simulink library "carnot"  (R2018b)
settings: Solver=VariableStepAuto  StartTime=0.0  StopTime=10.0  RelTol=1e-3
undefined symbols (not defined in the file or in its folder): A, A_earth, acol, Acol, ActPower1, ActPower2, ActPower3, Ad, Ad0, Ar, Au, Au0, Azimuth_Angle, B, Bd, Bd0, Br, Bu, Bu0, C, c1, c2, c3, c33, c4, c5, c6, CarnotCallbacks_Density, CarnotCallbacks_Enthalpy, CarnotCallbacks_Enthalpy2Temperature, CarnotCallbacks_Entropy, CarnotCallbacks_Evaporation_Enthalpy, CarnotCallbacks_GlobalMessageLevel, CarnotCallbacks_Grashof, CarnotCallbacks_Heat_Capacity, CarnotCallbacks_Kinematic_Viscosity, CarnotCallbacks_PMV_PPD, CarnotCallbacks_Prandtl, CarnotCallbacks_Saturation_Property, CarnotCallbacks_Saturation_Temperature, CarnotCallbacks_Saturation_Value_Water, CarnotCallbacks_Specific_Volume, CarnotCallbacks_Thermal_Conductivity, CarnotCallbacks_Vapour_Content, CarnotCallbacks_Vapour_Pressure, Cd, Cdl, Cr, Cu, Davies, Dd, DE_TRY2010_04_averageYear, delta_grd, density, DiameterLastPiece, dl, DPConstant, DPLinear, DPQuadratic, Dr ... (+59)
libraries: $bdroot x429, simulink x36, simulink_extras x12
(part 17 of 22)

== system carnot/Source/Solar_Thermal/IncidenceAngleModifier ==
  IAM_Table : Subsystem  mask(IAM Table for Solar Thermal Collectors){fta=0.8, angle=[0:5:90], Kb=[1.0000    1.0000    0.9999    0.9996    0.9991    0.9982    0.9965  0.9935    0.9886    0.9807    0.9678    0.9473    0.9148    0.8638   0.7846    0.6644    0.4907    0.2599    0.0000], Kd=0.92}
      mask prompts: fta "Fin Efficiency * Transmission * Absorption (FTA) [-]"; angle "Direct incidence angles for IAM [degree]"; Kb "Kdir: Incidence angle modifier direct radiation (0..1)"; Kd "Kdfu : Incidence angle modifier diffuse radiation"
      mask help:
      | Transforms direct and diffuse radiation to an absorbed solar power per unit area. The direct radiation incidence angle modifier (Kdir) uses the table-model for collectors (EN 12975).
      | FTA or F'(TauAlfa) is defined from the incidence angle modifiers Kdir and Kdfu:
      | FTA = eta0 / (Kdir(15°)*0.85 + Kdfu*0.15)
      | Direct radiation: Kdir and the incidence angle are vectors
      | Diffuse radiation  Kdfu = constant (at 50° incidence)
      mask Help: web(fullfile(path_carnot('help'),'IAM_Table.html'),'-helpbrowser')
  IAM_Table_KbL_KbT : Subsystem  mask(IAM Table for EN 12975 Solar Thermal Collector Model){fta=0.8, kblangle=[0:5:90], KbL=[1.0000    1.0000    0.9999    0.9996    0.9991    0.9982    0.9965  0.9935    0.9886    0.9807    0.9678    0.9473    0.9148    0.8638   0.7846    0.6644    0.4907    0.2599    0.0000], kbtangle=[0:5:90], KbT=[1.00000 1.00000 1.00000 1.00000 1.00000 1.00000 1.00000 1.00000 1.00000 1.00000 1.00000 0.87500 0.75000 0.62500 0.50000 0.37500 0.25000 0.12500 0], Kd=0.92}
      mask prompts: fta "Fin Efficiency * Transmission * Absorption (F'(tau alfa))"; kblangle "KbL: angles for longitudinal IAM [degree]"; KbL "KbL: values for longitudinal incidence angle modifier (0..1)"; kbtangle "KbT: angles for transversal IAM [degree]"; KbT "KbT: values for transversal incidence angle modifier (0..1)"; Kd "Kd : Incidence angle modifier diffuse radiation"
      mask help:
      | USE IN THE "Collector_EN12975" MODEL:
      | Transforms direct and diffuse radiation to an absorbed solar power per unit area. The direct radiation incidence angle modifier (Kdir) uses the b0-model for flat plate collectors (EN 12975).
      | FTA or F'(TauAlfa) is defined from the incidence angle modifiers Kdir and Kdfu:
      | FTA = eta0 / (Kdir(15°)*0.85 + Kdfu*0.15)
      | The direct radiation is split in a transversal (T) and longitudinal (L) component.
      | Direct radiation: Kb(L) and Kb(T) is given in an vecorized form
      | Diffuse radiation  Kd = constant (at 50° incidence)
      mask Help: web(fullfile(path_carnot('help'),'IAM_Table_KbL_KbT.html'),'-helpbrowser')
  IAM_b0 : Subsystem  mask(collector optics single glazing with extra white glass){fta=0.8, b0=0.12, Kd=0.92}
      mask prompts: fta "Fin Efficiency * Transmission * Absorption (FTA) [-]"; b0 "b0 : constant for the calculation of the incident angle modifier (direct radiation) [-]"; Kd "Kd : Incidence angle modifier diffuse radiation [-]"
      mask help:
      | USE IN THE "Collector_EN12975_FlatPlate" MODEL:
      | Transforms direct and diffuse radiation to an absorbed solar power per unit area. The direct radiation incidence angle modifier (Kdir) uses the b0-model for flat plate collectors (EN 12975).
      | FTA or F'(TauAlfa) is defined from the incidence angle modifiers Kdir and Kdfu:
      | FTA = eta0 / (Kdir(15°)*0.85 + Kdfu*0.15)
      mask Help: web(fullfile(path_carnot('help'),'IAM_b0.html'),'-helpbrowser')
  Theoretical_Collector_Optics : Subsystem  mask(theoretical collector optics){FTA=0.8, ncover=1, refin=1.525, d=0.004, ext=4}
      mask prompts: FTA "Fin Efficiency * Transmission * Absorption (FTA) [-]"; ncover "Number of covers [-]"; refin "Refraction index of material [-]"; d "Thickness of the material in m"; ext "Extinction coefficient in 1/m"
      mask help:
      | Transforms direct and diffuse radiation to an absorbed solar power per unit area. FTA or F'(TauAlfa) is defined from the incidence angle modifiers Kdir and Kdfu:
      | FTA = eta0 / (Kdir(15°)*0.85 + Kdfu*0.15)
      | Kdir (for direct radiation) and Kdfu (for diffuse radiation) are derived from Fresnels equations refraction index (glass = 1.526), the thickness and the extinction coefficient (extra white glass 4/m, float glass 16/m).
      | See "taualfa" in the manual or type "help taualfa" on the command line for more information on the calculation of the IAM.
      mask init:
      | teta = [0:5:90]; % incidence angle
      | KL = d*ext; % extiction * thickness
      | kb = taualfa (ncover, refin, teta*pi/180, KL, 1);
      | kd = taualfa (ncover, refin, pi/3, KL, 1);
      | kd = kd/kb(1);
      | kb = kb/kb(1);
      mask Help: web(fullfile(path_carnot('help'),'Theoretical_Collector_Optics.html'),'-helpbrowser')

== system carnot/Source/Solar_Thermal/PressureDropCollector ==
  pressure_drop_calculated_data_water : Subsystem  mask(pressure drop for header - riser, fluid water){aonecol=1.96, acol=acol}
      mask prompts: aonecol "surface of one collector element [m²]"; acol "total surface of array (DO NOT CHANGE)"
      mask help:
      | This block interpolates the pressure drop of a collector for a usual header riser- arrangement. The number of risers (= number of absorber fins) is 10 per m². The inner diameter of the riser is 6 mm, of the header 20 mm. Fluid in the collector is water. An equation of Dunkle and Davey ("Flow distribution in absorber banks", ISES Conference, 1970) is used. See colpdrop in the manual or type "help colpdrop" on the command line for more information.
      | Set "surface of one collector" to the surface of one collector for a parallel arrangement of collectors. Set it to the surface of the array "acol" to model a series arrangement.
      mask Help: web(fullfile(path_carnot('help'),'pressure_drop_calculated_for_header_riser_water.html'),'-helpbrowser')
  pressure_drop_for_measured_data_water : Subsystem  mask(pressure drop measured data, fluid water){mdottest=0.01*1.96, ttest=20, pdroptest=158*1.96, aonecol=1.96, acol=acol}
      mask prompts: mdottest "massflow at test condition condition [kg/s]"; ttest "temperature at test condition [degree centigrade]"; pdroptest "pressure drop in test [Pa]"; aonecol "surface of one collector [m²]"; acol "total surface of array (DO NOT CHANGE HERE)"
      mask help:
      | This block calculates the pressure drop of a collector from measured data.
      | Other massflow rates and temperatures than at test condition are interpolated according to a typical massflow to pressure drop correlation of a collector for the fluid water.
      | Set "surface of one collector" to the surface of one collector for a parallel arrangement of collectors. Set it to the surface of the array "acol" to model a series arrangement.
      mask Help: web(fullfile(path_carnot('help'),'pressure_drop_for_measured_data_water.html'),'-helpbrowser')
  pressure_drop_quadratic_fitted_data : Subsystem  mask(pressure drop quadratic fitted data, fluid water){b=0.006201*3.6e4, a=0.000096*1.296e9, aonecol=1.96, acol=acol}
      mask prompts: b "linear term of pressure drop in [Pa/(kg/s)]"; a "quadratic term of pressure drop in [Pa/(kg/s)²]"; aonecol "surface of one collector element in [m²]"; acol "total surface of array (DO NOT CHANGE HERE)"
      mask help:
      | This block calculates the pressure drop of a collector from a fitted parabolic curve. Other temperatures than at test condition are not corrected.
      | Give parameters in SI-units.
      | Multiply with 3.6e5 to convert from [mbar/(l/h)] to [Pa/(kg/s)].
      | Multiply with 1.296e9 to convert from [mbar/(l/h)²] to [Pa/(kg/s)²].
      | Set "surface of one collector" to the surface of one collector for a parallel arrangement of collectors. Set it to the surface of the array "acol" to model a series arrangement.
      mask Help: web(fullfile(path_carnot('help'),'pressure_drop_quadratic_fitted_data.html'),'-helpbrowser')
  pressure_drop_quadratic_fitted_data_water : Subsystem  mask(pressure drop quadratic fitted data, fluid water){b=0.006201*3.6e4, a=0.000096*1.296e9, aonecol=1.96, acol=acol}
      mask prompts: b "linear term of pressure drop in [Pa/(kg/s)]"; a "quadratic term of pressure drop in [Pa/(kg/s)²]"; aonecol "surface of one collector element in [m²]"; acol "total surface of array (DO NOT CHANGE HERE)"
      mask help:
      | This block calculates the pressure drop of a collector from a fitted parabolic curve. Other temperatures than at test condition (20°C) are interpolated according to a typical pressure drop correlation of a collector for the fluid water.
      | Give parameters in SI-units.
      | Multiply with 3.6e5 to convert from [mbar/(l/h)] to [Pa/(kg/s)].
      | Multiply with 1.296e9 to convert from [mbar/(l/h)²] to [Pa/(kg/s)²].
      | Set "surface of one collector" to the surface of one collector for a parallel arrangement of collectors. Set it to the surface of the array "acol" to model a series arrangement.
      mask Help: web(fullfile(path_carnot('help'),'pressure_drop_quadratic_fitted_data_water.html'),'-helpbrowser')

== system carnot/Source/Solar_Thermal/SolarCollector ==
  WDB : Inport
  position : Inport  Port=2
  THBin : Inport  Port=3
  Acol : Constant  Value=acol
  Bus Assignment : BusAssignment  AssignedSignals=MassFlow
  Bus Assignment1 : BusAssignment  AssignedSignals=MassFlow
  Bus Selector : BusSelector  OutputSignals=MassFlow
  Divide : Product  Inputs=/*
  Gain1 : Gain  Gain=Ncollector
  Gain2 : Gain  Gain=Ncollector
  Ncollector : Constant  Value=Ncollector
  Pressure_Drop_Collector : $bdroot/Basic/Pressure_Drop/Pressure_Drop_Collector  len=len  lin=dplin  qua=dpqua
  Radiation_on_Inclined_Surface : $bdroot/Weather/Radiation_on_Inclined_Surface  sky=Perez 1990  reflect=0.2
  T_Sensor : $bdroot/Control/T_Sensor  tc=SensorTimeConstant  t0=t0
  create_Cdat : Subsystem
  glazed_collector_ISO9806 : Subsystem  mask(Basic Solar Thermal Collector){acol=acol, fta=fta, c1=c1, c2=c2, c3=c3, c4=c4, c5=c5, c6=c6, tini=t0, kblangle=KbAngles, KbL=KbL, kbtangle=KbAngles, KbT=KbT, Kd=Kd}
      mask prompts: acol "A : collector surface  [m²]"; fta "Fin Efficiency * Transmission * Absorption (F'(tau alfa))"; c1 "c1 : heat loss coefficient at (Tm-Ta)=0  [W/(m²*K)]"; c2 "c2: temperature dependence of the heat loss coefficient [W/(m*K)²]"; c3 "c3 : wind speed dependence of the heat loss coefficient [J/(m³K)]"; c4 "c4 : sky temperature dependence of the heat loss coefficient [W/(m²K)]"; c5 "c5 : effective thermal capacity [J/(m²K)]"; c6 "c6 : wind dependence in the zero loss efficiency [s/m]"; tini "initial temperature [degree Celsius]"; kblangle "KbL: angles for longitudinal IAM [degree]"; KbL "KbL: values for longitudinal incidence angle modifier (0..1)"; kbtangle "KbT: angles for transversal IAM [degree]"; KbT "KbT: values for transversal incidence angle modifier (0..1)"; Kd "Kd : Incidence angle modifier diffuse radiation"
      mask help: Model according to EN 12975 / ISO 22975
      mask Help: web(fullfile(path_carnot('help'),'Solar_Collector_basic.html'),'-helpbrowser')
      mask TypeOptions fta: IAM_Table_KbL_KbT/fta
      mask TypeOptions kblangle: IAM_Table_KbL_KbT/kblangle
      mask TypeOptions KbL: IAM_Table_KbL_KbT/KbL
      mask TypeOptions kbtangle: IAM_Table_KbL_KbT/kbtangle
      mask TypeOptions KbT: IAM_Table_KbL_KbT/KbT
      mask TypeOptions Kd: IAM_Table_KbL_KbT/Kd
      mask DialogControl Container4 Prompt: Collector Parameters
      mask DialogControl Container10 Prompt: Optics
      mask Display: disp('glazed\nsolar\nthermal\ncollector\nISO 9806')
  Cdat : Outport
  Tsol : Outport  Port=2
  THB : Outport  Port=3
  wires:
  Bus Assignment1/1 -> T_Sensor/1
  Gain2/1 -> create_Cdat/4(Qdot)
  Gain1/1 -> create_Cdat/1(acol)
  Bus Selector/1 -> Divide/2, Bus Assignment1/2  "<MassFlow>"
  Acol/1 -> Gain1/1
  position/1 -> Radiation_on_Inclined_Surface/2, Pressure_Drop_Collector/3
  Pressure_Drop_Collector/1 -> Bus Assignment1/1, create_Cdat/3(THBout)  "THB_s"
  Radiation_on_Inclined_Surface/1 -> create_Cdat/6(WDB), glazed_collector_ISO9806/1(WDB_surface)  "WDB_surface"
  create_Cdat/1(Cdat) -> Cdat/1  "Cdat"
  glazed_collector_ISO9806/2(Tm) -> create_Cdat/5(Tmean), Pressure_Drop_Collector/1  "Tmean"
  THBin/1 -> Bus Assignment/1, create_Cdat/2(THBin), Bus Selector/1  "THBin"
  glazed_collector_ISO9806/3(THB) -> Pressure_Drop_Collector/2  "THBout"
  glazed_collector_ISO9806/1(Qdot) -> Gain2/1  "Qdot"
  WDB/1 -> Radiation_on_Inclined_Surface/1
  Ncollector/1 -> Divide/1
  Divide/1 -> Bus Assignment/2
  T_Sensor/2 -> Tsol/1  "Tsol"
  T_Sensor/1 -> THB/1  "THB"
  Bus Assignment/1 -> glazed_collector_ISO9806/2(THBin)

== system carnot/Source/Solar_Thermal/SolarCollector_2node ==
  WDB : Inport
  position : Inport  Port=2
  THBin : Inport  Port=3
  Acol : Constant  Value=acol
  Bus Assignment : BusAssignment  AssignedSignals=MassFlow
  Bus Assignment1 : BusAssignment  AssignedSignals=MassFlow
  Bus Selector : BusSelector  OutputSignals=MassFlow
  Divide : Product  Inputs=/*
  Gain1 : Gain  Gain=Ncollector
  Gain2 : Gain  Gain=Ncollector
  Ncollector : Constant  Value=Ncollector
  Pressure_Drop_Collector : $bdroot/Basic/Pressure_Drop/Pressure_Drop_Collector  len=len  lin=dplin  qua=dpqua
  Radiation_on_Inclined_Surface : $bdroot/Weather/Radiation_on_Inclined_Surface  sky=Perez 1990  reflect=0.2
  T_Sensor : $bdroot/Control/T_Sensor  tc=SensorTimeConstant  t0=t0
  create_Cdat : Subsystem
  glazed_collector_ISO9806 : Subsystem  mask(Basic Solar Thermal Collector){acol=acol, fta=fta, c1=c1, c2=c2, c3=c3, c4=c4, c5=c5, c6=c6, tini=t0, kblangle=KbAngles, KbL=KbL, kbtangle=KbAngles, KbT=KbT, Kd=Kd}
      mask prompts: acol "A : collector surface  [m²]"; fta "Fin Efficiency * Transmission * Absorption (F'(tau alfa))"; c1 "c1 : heat loss coefficient at (Tm-Ta)=0  [W/(m²*K)]"; c2 "c2: temperature dependence of the heat loss coefficient [W/(m*K)²]"; c3 "c3 : wind speed dependence of the heat loss coefficient [J/(m³K)]"; c4 "c4 : sky temperature dependence of the heat loss coefficient [W/(m²K)]"; c5 "c5 : effective thermal capacity [J/(m²K)]"; c6 "c6 : wind dependence in the zero loss efficiency [s/m]"; tini "initial temperature [degree Celsius]"; kblangle "KbL: angles for longitudinal IAM [degree]"; KbL "KbL: values for longitudinal incidence angle modifier (0..1)"; kbtangle "KbT: angles for transversal IAM [degree]"; KbT "KbT: values for transversal incidence angle modifier (0..1)"; Kd "Kd : Incidence angle modifier diffuse radiation"
      mask help: Model according to EN 12975 / ISO 22975
      mask Help: web(fullfile(path_carnot('help'),'Solar_Collector_basic.html'),'-helpbrowser')
      mask TypeOptions fta: IAM_Table_KbL_KbT/fta
      mask TypeOptions kblangle: IAM_Table_KbL_KbT/kblangle
      mask TypeOptions KbL: IAM_Table_KbL_KbT/KbL
      mask TypeOptions kbtangle: IAM_Table_KbL_KbT/kbtangle
      mask TypeOptions KbT: IAM_Table_KbL_KbT/KbT
      mask TypeOptions Kd: IAM_Table_KbL_KbT/Kd
      mask DialogControl Container4 Prompt: Collector Parameters
      mask DialogControl Container10 Prompt: Optics
      mask Display: disp('glazed\nsolar\nthermal\ncollector\nISO 9806')
  Cdat : Outport
  Tsol : Outport  Port=2
  THB : Outport  Port=3
  wires:
  Bus Assignment1/1 -> T_Sensor/1
  Gain2/1 -> create_Cdat/4(Qdot)
  Gain1/1 -> create_Cdat/1(acol)
  Bus Selector/1 -> Divide/2, Bus Assignment1/2  "<MassFlow>"
  Acol/1 -> glazed_collector_ISO9806/2(Acol), Gain1/1
  position/1 -> Radiation_on_Inclined_Surface/2, Pressure_Drop_Collector/3
  Pressure_Drop_Collector/1 -> create_Cdat/3(THBout), Bus Assignment1/1  "THB_s"
  Radiation_on_Inclined_Surface/1 -> glazed_collector_ISO9806/1(WDB_surface), create_Cdat/6(WDB)  "WDB_surface"
  create_Cdat/1(Cdat) -> Cdat/1  "Cdat"
  glazed_collector_ISO9806/2(Tm) -> Pressure_Drop_Collector/1, create_Cdat/5(Tmean)  "Tmean"
  THBin/1 -> Bus Assignment/1, create_Cdat/2(THBin), Bus Selector/1  "THBin"
  glazed_collector_ISO9806/3(THB) -> Pressure_Drop_Collector/2  "THBout"
  glazed_collector_ISO9806/1(qdot) -> Gain2/1
  WDB/1 -> Radiation_on_Inclined_Surface/1
  Ncollector/1 -> Divide/1
  Divide/1 -> Bus Assignment/2
  T_Sensor/2 -> Tsol/1  "Tsol"
  T_Sensor/1 -> THB/1  "THB"
  Bus Assignment/1 -> glazed_collector_ISO9806/3(THBin)

== system carnot/Source/Ventilation/Constant_AIV ==
  const : Constant  Value=[Tsens Tcon Trad mw mco rhoair cpair pair nair]
  AIV_out : Outport
  wires:
  const/1 -> AIV_out/1

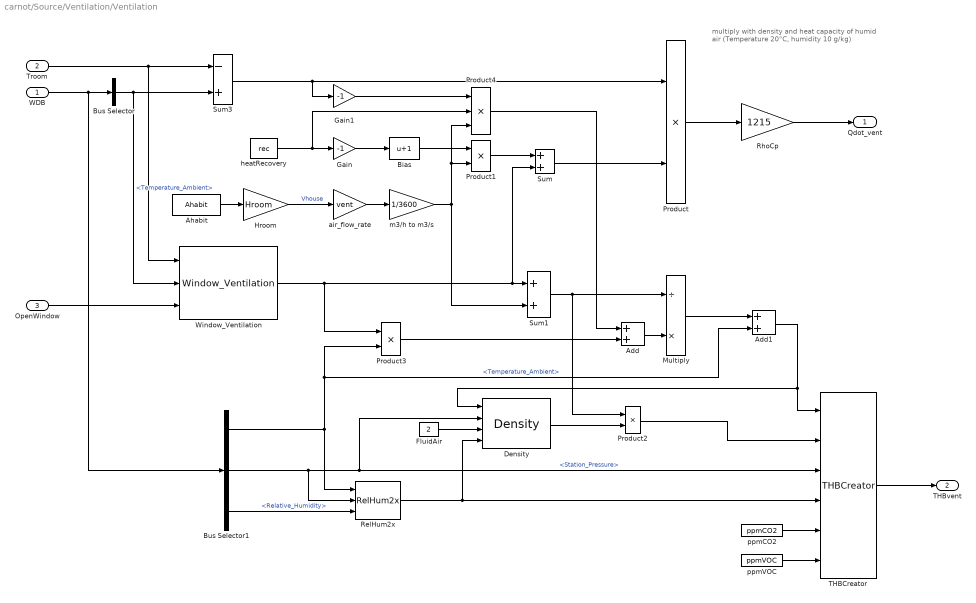
== system carnot/Source/Ventilation/Ventilation ==
  note: multiply with density and
      | heat capacity of humid air
      | (Temperature 20°C, humidity 10 g/kg)
  WDB : Inport
  Troom : Inport  Port=2
  OpenWindow : Inport  Port=3
  Add : Sum
  Add1 : Sum
  Ahabit : Constant  Value=Ahabit
  Bias : Bias  Bias=1
  Bus Selector : BusSelector  OutputSignals=Temperature_Ambient
  Bus Selector1 : BusSelector  OutputSignals=Temperature_Ambient,Station_Pressure,Relative_Humidity
  Density : $bdroot/Basic/Material_Properties/Density  VariantControl=CarlibClassic  INPUTARGUMENTS=state variables (classic)  DEBUGLEVEL=DEBUGLEVEL  MAXTOTALWARNINGS=inf  MAXCONSECUTIVEWARNINGS=inf  WRITETOFILE=0  FILENAME='errors.txt'
  FluidAir : Constant  Value=2
  Gain : Gain  Gain=-1
  Gain1 : Gain  Gain=-1
  Hroom : Gain  Gain=Hroom
  Multiply : Product  Inputs=/*
  Product : Product  RndMeth=Zero
  Product1 : Product  Inputs=**  RndMeth=Zero
  Product2 : Product  RndMeth=Zero
  Product3 : Product  RndMeth=Zero
  Product4 : Product  Inputs=3  RndMeth=Zero
  RelHum2x : $bdroot/Basic/Material_Properties/RelHum2x
  RhoCp : Gain  Gain=1215  SaturateOnIntegerOverflow=on  OutDataTypeStr=Inherit: Same as input  ParamDataTypeStr=Inherit: Same as input
  Sum : Sum
  Sum1 : Sum
  Sum3 : Sum  Inputs=-+  SaturateOnIntegerOverflow=on  InputSameDT=on  OutDataTypeStr=Inherit: Same as first input
  THBCreator : $bdroot/Basic/Hydraulics/THBCreator  Inport_ID=off  Inport_T=on  Inport_mdot=on  Inport_p=on  Inport_type=off  Inport_mix=on  Inport_mix2=on  Inport_mix3=on  Inport_d=off  Inport_c=off  Inport_l=off  Inport_q=off  Inport_LH=off  Inport_H=off  ID=1  T=20  mdot=0  p=1e5  FluidType=2  FluidMix=0  FluidMix2=0  FluidMix3=0  d=1  c=0  l=0  q=0  LH=1  H=0  Annotation_ID=off  Annotation_T=off  Annotation_mdot=off  Annotation_p=off  Annotation_type=off  Annotation_mix=off  Annotation_mix2=off  Annotation_mix3=off  Annotation_d=off  Annotation_c=off  Annotation_l=off  Annotation_q=off  Annotation_LH=off  Annotation_H=off
  Window_Ventilation : $bdroot/Source/Ventilation/Window_Ventilation  alpha=alpha  H=H  W=W  Nwin=Nwin
  air_flow_rate : Gain  Gain=vent
  heatRecovery : Constant  Value=rec
  m3/h to m3/s : Gain  Gain=1/3600  SaturateOnIntegerOverflow=on  OutDataTypeStr=Inherit: Same as input  ParamDataTypeStr=Inherit: Same as input
  ppmCO2 : Constant  Value=ppmCO2
  ppmVOC : Constant  Value=ppmVOC
  Qdot_vent : Outport
  THBvent : Outport  Port=2
  wires:
  Gain1/1 -> Product4/1
  Add1/1 -> Density/1, THBCreator/1
  Multiply/1 -> Add1/1
  Add/1 -> Multiply/2
  Product4/1 -> Add/1
  Sum3/1 -> Gain1/1, Product/1
  Product3/1 -> Add/2
  Sum1/1 -> Multiply/1, Product2/1
  Bias/1 -> Product1/1
  Product1/1 -> Sum/1
  RhoCp/1 -> Qdot_vent/1
  Window_Ventilation/1 -> Sum/2, Sum1/1, Product3/1
  FluidAir/1 -> Density/3
  Density/1 -> Product2/2
  air_flow_rate/1 -> m3/h to m3/s/1
  Product2/1 -> THBCreator/2
  ppmVOC/1 -> THBCreator/6
  ppmCO2/1 -> THBCreator/5
  RelHum2x/1 -> Density/4, THBCreator/4
  Bus Selector1/3 -> RelHum2x/3  "<Relative_Humidity>"
  Bus Selector1/2 -> RelHum2x/2, Density/2, THBCreator/3  "<Station_Pressure>"
  Bus Selector1/1 -> RelHum2x/1, Product3/2, Add1/2  "<Temperature_Ambient>"
  Bus Selector/1 -> Window_Ventilation/2, Sum3/2  "<Temperature_Ambient>"
  THBCreator/1 -> THBvent/1
  Sum/1 -> Product/2
  Product/1 -> RhoCp/1
  Ahabit/1 -> Hroom/1
  Hroom/1 -> air_flow_rate/1  "Vhouse"
  WDB/1 -> Bus Selector1/1, Bus Selector/1
  m3/h to m3/s/1 -> Product1/2, Product4/3, Sum1/2
  Troom/1 -> Sum3/1, Window_Ventilation/1
  OpenWindow/1 -> Window_Ventilation/3
  heatRecovery/1 -> Gain/1, Product4/2
  Gain/1 -> Bias/1

== system carnot/Source/Ventilation/Ventilation_AIV ==
  note: ASSUMPTION: Vdot_air_in = Vdot_air_out !
  note: AIR VENTILATION outdoors - indoors
  air_exchange_rate : Inport
  "[AIV]" : Inport  Port=2
  WDB : Inport  Port=3
  Vair : Inport  Port=4
  "\"air\"" : Constant  Value=2
  "1/h -> 1/s" : Gain  Gain=1/3600  SaturateOnIntegerOverflow=on  OutDataTypeStr=Inherit: Same as input  ParamDataTypeStr=Inherit: Same as input
  Bus Selector : BusSelector  OutputSignals=Temperature_Ambient,Relative_Humidity,Station_Pressure
  Constant{,1..5} (6 alike) : Constant  Value=0
  Demux2 : Demux  Outputs=[1 1 1 2 4]
  Density : $bdroot/Basic/Material_Properties/Density  VariantControl=CarlibClassic  INPUTARGUMENTS=state variables (classic)  DEBUGLEVEL=DEBUGLEVEL  MAXTOTALWARNINGS=inf  MAXCONSECUTIVEWARNINGS=inf  WRITETOFILE=0  FILENAME='errors.txt'
  Heat_Capacity : $bdroot/Basic/Material_Properties/Heat_Capacity  VariantControl=CarlibClassic  INPUTARGUMENTS=state variables (classic)  DEBUGLEVEL=DEBUGLEVEL  MAXTOTALWARNINGS=inf  MAXCONSECUTIVEWARNINGS=inf  WRITETOFILE=0  FILENAME='errors.txt'
  Mux : Mux  Inputs=1
  Mux1 : Mux  Inputs=13
  Mux2 : Mux  Inputs=1
  Mux4 : Mux  Inputs=2
  Product1 : Product  SaturateOnIntegerOverflow=on  InputSameDT=on  OutDataTypeStr=Inherit: Same as first input
  Product2 : Product  SaturateOnIntegerOverflow=on  InputSameDT=on  OutDataTypeStr=Inherit: Same as first input
  Product4 : Product  Inputs=3  SaturateOnIntegerOverflow=on  InputSameDT=on  OutDataTypeStr=Inherit: Same as first input
  RelHum2x : $bdroot/Basic/Material_Properties/RelHum2x
  Saturation : Saturate  UpperLimit=inf  LowerLimit=0
  Subsystem : Subsystem
  Sum : Sum  Inputs=-+  SaturateOnIntegerOverflow=on  InputSameDT=on  OutDataTypeStr=Inherit: Same as first input
  Terminator : Terminator
  Terminator1 : Terminator
  Terminator2 : Terminator
  rho(CO2) / rho(air) * CO2norm (kg/kg) : Constant  Value=1.529*CO2norm
  "[S]" : Outport
  wires:
  Constant5/1 -> Mux1/8  "Qdotr"
  Mux2/1 -> Mux1/7  "Qdotc"
  Mux1/1 -> "[S]"/1
  Constant/1 -> Mux1/1  "Qdot_sol"
  Constant1/1 -> Mux1/2  "Qdot_equip"
  Constant2/1 -> Mux1/3  "Qdot_light"
  Constant3/1 -> Mux1/4  "Qdot_pers"
  Constant4/1 -> Mux1/5  "Qdot_heat"
  Mux/1 -> Mux1/13  "Vdot_in2out"
  "1/h -> 1/s"/1 -> Product1/1
  Vair/1 -> Product1/2
  Product4/1 -> Mux1/6, Mux2/1  "Qdot_air"
  Subsystem/3(D_mdot_CO2) -> Mux1/11  "D_mdot_CO2"
  Subsystem/2(D_mdot_H2O) -> Mux1/10  "D_mdot_H2O"
  WDB/1 -> Bus Selector/1
  air_exchange_rate/1 -> Saturation/1
  "[AIV]"/1 -> Demux2/1
  Density/1 -> Product2/2
  Bus Selector/3 -> Heat_Capacity/2, Density/2, RelHum2x/2  "<Station_Pressure>"
  Bus Selector/2 -> RelHum2x/3  "<Relative_Humidity>"
  Bus Selector/1 -> RelHum2x/1, Heat_Capacity/1, Sum/2, Density/1  "<Temperature_Ambient>"
  RelHum2x/1 -> Heat_Capacity/4, Density/4, Mux4/1  "x_H2O"
  "\"air\""/1 -> Density/3, Heat_Capacity/3
  Demux2/4 -> Subsystem/2(x_in)  "[x_H2O, x_CO2]_in"
  Demux2/5 -> Terminator2/1
  Demux2/3 -> Terminator1/1
  Demux2/2 -> Sum/1  "Tc"
  Mux4/1 -> Subsystem/3(x_out)
  rho(CO2) / rho(air) * CO2norm (kg/kg)/1 -> Mux4/2  "x_CO2"
  Sum/1 -> Product4/1  "dT"
  Demux2/1 -> Terminator/1
  Heat_Capacity/1 -> Product4/2  "cp"
  Product2/1 -> Product4/3, Subsystem/1(mdot_air)  "mdot_air"
  Saturation/1 -> "1/h -> 1/s"/1
  Product1/1 -> Mux1/12, Mux/1, Product2/1  "Vdot_out2in"
  Subsystem/1(D_mdot_air) -> Mux1/9  "D_mdot_air"

== system carnot/Source/Ventilation/Window_Ventilation ==
  note: range is 0 to 1
  Troom : Inport
  Tamb : Inport  Port=2
  Ctrl : Inport  Port=3
  Mux : Mux  Inputs=3
  NumberOfWindows : Gain  Gain=Nwin
  S-Function : S-Function  FunctionName=tiltvent  Parameters=alpha, H, W  SFunctionDeploymentMode=off  EnableBusSupport=off
  Saturation : Saturate  UpperLimit=1  LowerLimit=0
  Vdot : Outport
  wires:
  Saturation/1 -> Mux/3
  Troom/1 -> Mux/1
  Mux/1 -> S-Function/1
  S-Function/1 -> NumberOfWindows/1
  Ctrl/1 -> Saturation/1
  Tamb/1 -> Mux/2
  NumberOfWindows/1 -> Vdot/1

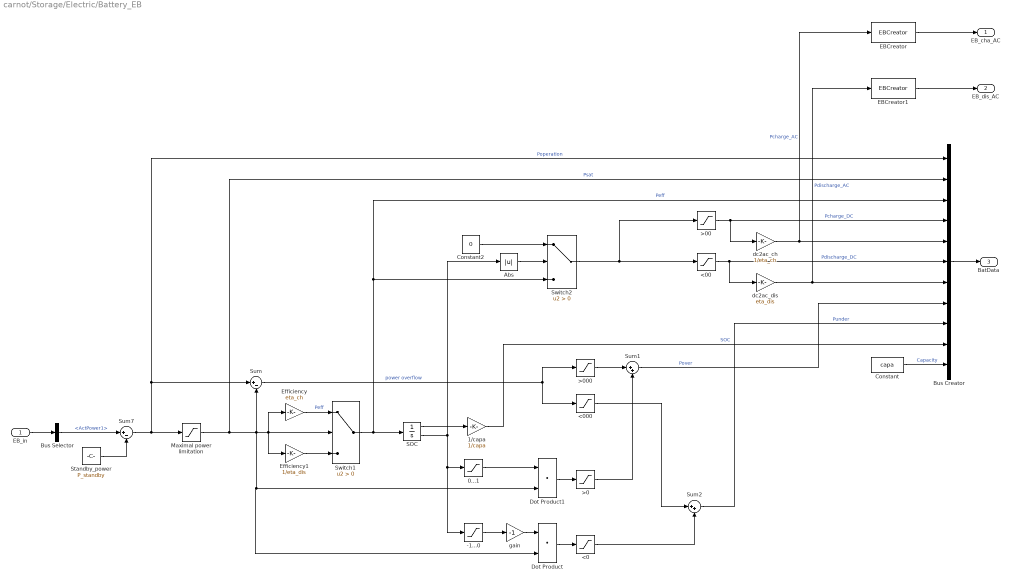
== system carnot/Storage/Electric/Battery_EB ==
  EB_in : Inport
  -1...0 : Saturate  UpperLimit=0  LowerLimit=-1
  0...1 : Saturate  UpperLimit=1  LowerLimit=0
  1/capa : Gain  Gain=1/capa
  <0 : Saturate  UpperLimit=0  LowerLimit=-inf
  <00 : Saturate  UpperLimit=0  LowerLimit=-inf
  <000 : Saturate  UpperLimit=0  LowerLimit=-inf
  >0 : Saturate  UpperLimit=inf  LowerLimit=0
  >00 : Saturate  UpperLimit=inf  LowerLimit=0
  >000 : Saturate  UpperLimit=inf  LowerLimit=0
  Abs : Abs
  Bus Creator : BusCreator  Inputs=11
  Bus Selector : BusSelector  OutputSignals=ActPower1
  Constant : Constant  Value=capa
  Constant2 : Constant  Value=0
  Dot Product : DotProduct  InputSameDT=on  OutDataTypeStr=Inherit: Inherit via internal rule
  Dot Product1 : DotProduct  InputSameDT=on  OutDataTypeStr=Inherit: Inherit via internal rule
  EBCreator : $bdroot/Basic/Electric/EBCreator  Inport_ID=off  Inport_f=off  Inport_v1=off  Inport_p1=on  Inport_pf1=off  Inport_v2=off  Inport_p2=off  Inport_pf2=off  Inport_v3=off  Inport_p3=off  Inport_pf3=off  ID=1  f=0  v1=400%dummy  p1=1e5  pf1=1  v2=0  p2=1e5  pf2=1  v3=0  p3=0  pf3=1  Annotation_ID=on  Annotation_f=on  Annotation_v1=on  Annotation_p1=off  Annotation_pf1=off  Annotation_v2=off  Annotation_p2=off  Annotation_pf2=off  Annotation_v3=off  Annotation_p3=off  Annotation_pf3=off
      settings: AttributesFormatString=|
      | ID 1
      | 0 Hz frequency
      | 400%dummy V Voltage
  EBCreator1 : $bdroot/Basic/Electric/EBCreator  Inport_ID=off  Inport_f=off  Inport_v1=off  Inport_p1=on  Inport_pf1=off  Inport_v2=off  Inport_p2=off  Inport_pf2=off  Inport_v3=off  Inport_p3=off  Inport_pf3=off  ID=1  f=0  v1=400%dummy  p1=1e5  pf1=1  v2=0  p2=1e5  pf2=1  v3=0  p3=0  pf3=1  Annotation_ID=on  Annotation_f=on  Annotation_v1=on  Annotation_p1=off  Annotation_pf1=off  Annotation_v2=off  Annotation_p2=off  Annotation_pf2=off  Annotation_v3=off  Annotation_p3=off  Annotation_pf3=off
      settings: AttributesFormatString=|
      | ID 1
      | 0 Hz frequency
      | 400%dummy V Voltage
  Efficiency : Gain  Gain=eta_ch
  Efficiency1 : Gain  Gain=1/eta_dis
  Maximal power limitation : Saturate  UpperLimit=Pmax/eta_ch  LowerLimit=-Pmin*eta_dis
  SOC : Integrator  InitialCondition=cap0*capa  LimitOutput=on  UpperSaturationLimit=SOC_max*capa  LowerSaturationLimit=SOC_min*capa  ShowSaturationPort=on
  Standby_power : Constant  Value=P_standby
  Sum : Sum  Inputs=|+-
  Sum1 : Sum  Inputs=|++
  Sum2 : Sum  Inputs=|++
  Sum7 : Sum  Inputs=|+-
  Switch1 : Switch  Criteria=u2 > Threshold
  Switch2 : Switch  Criteria=u2 > Threshold
  dc2ac_ch : Gain  Gain=1/eta_ch
  dc2ac_dis : Gain  Gain=eta_dis
  gain : Gain  Gain=-1
  EB_cha_AC : Outport
  EB_dis_AC : Outport  Port=2
  BatData : Outport  Port=3
  wires:
  EBCreator/1 -> EB_cha_AC/1
  EBCreator1/1 -> EB_dis_AC/1
  dc2ac_dis/1 -> Bus Creator/7, EBCreator1/1  "Pdischarge_AC"
  dc2ac_ch/1 -> Bus Creator/5, EBCreator/1  "Pcharge_AC"
  Sum1/1 -> Bus Creator/8  "Pover"
  Sum7/1 -> Bus Creator/1, Sum/1, Maximal power limitation/1  "Poperation"
  Constant2/1 -> Switch2/1
  Abs/1 -> Switch2/2
  Switch2/1 -> >00/1, <00/1
  Efficiency1/1 -> Switch1/3
  Efficiency/1 -> Switch1/1  "Peff"
  Standby_power/1 -> Sum7/2
  Switch1/1 -> Bus Creator/3, Switch2/3, SOC/1  "Peff"
  Dot Product1/1 -> >0/1
  0...1/1 -> Dot Product1/1
  -1...0/1 -> gain/1
  Dot Product/1 -> <0/1
  gain/1 -> Dot Product/1
  SOC/2 -> -1...0/1, 0...1/1, Abs/1
  1/capa/1 -> Bus Creator/10  "SOC"
  SOC/1 -> 1/capa/1
  Maximal power limitation/1 -> Bus Creator/2, Efficiency/1, Efficiency1/1, Switch1/2, Dot Product1/2, Dot Product/2, Sum/2  "Psat"
  Sum/1 -> >000/1, <000/1  "power overflow"
  >0/1 -> Sum1/2
  >000/1 -> Sum1/1
  <0/1 -> Sum2/2
  <000/1 -> Sum2/1
  <00/1 -> Bus Creator/6, dc2ac_dis/1  "Pdischarge_DC"
  Bus Creator/1 -> BatData/1
  Sum2/1 -> Bus Creator/9  "Punder"
  >00/1 -> Bus Creator/4, dc2ac_ch/1  "Pcharge_DC"
  EB_in/1 -> Bus Selector/1
  Bus Selector/1 -> Sum7/1  "<ActPower1>"
  Constant/1 -> Bus Creator/11  "Capacity"

== system carnot/Storage/Thermal/Ground_Storage ==
  WDB : Inport
  T_top : Inport  Port=2
  THVin : Inport  Port=3
  Tsurface : Inport  Port=4
  Tbottom : Inport  Port=5
  Demux : Demux  Outputs=[3*mpts 1 1 3]
  Demux1 : Demux  Outputs=[1 1 1 1 2 4]
  Demux2 : Demux  Outputs=[10 10]
  Isolated_Cover : $bdroot/Storage/Thermal/surface_models/Isolated_Cover  u=0.6
  Mux : Mux  Inputs=10
  Mux1 : Mux  Inputs=8
  Open_Surface : $bdroot/Storage/Thermal/surface_models/Open_Surface  albedo=0.6
  S-Function : S-Function  FunctionName=ground  Parameters=xs, ys, zs, cg, lg, dp, kp, np, zp, cf, lf, t0, refine, mpts  SFunctionDeploymentMode=off  EnableBusSupport=off
  diameter : Constant  Value=dp
  THV : Outport
  Tnodes : Outport  Port=2
  wires:
  T_top/1 -> Isolated_Cover/1
  S-Function/1 -> Demux/1
  Demux1/1 -> Mux/3, Mux1/1  "ID"
  Isolated_Cover/1 -> Mux/2
  Open_Surface/1 -> Mux/1
  WDB/1 -> Open_Surface/1
  diameter/1 -> Mux1/6
  Mux/1 -> S-Function/1
  Demux/3 -> Mux1/4  "p"
  Demux/2 -> Mux1/2  "T"
  Mux1/1 -> THV/1
  Demux/1 -> Tnodes/1
  Tbottom/1 -> Mux/10
  Tsurface/1 -> Mux/9
  Demux1/5 -> Mux1/5, Mux/7  "fluid, mix"
  Demux1/3 -> Mux1/3, Mux/5  "mdot"
  Demux1/6 -> Mux/8  "d clq"
  Demux1/4 -> Mux/6  "p"
  Demux1/2 -> Mux/4  "T"
  THVin/1 -> Demux2/1
  Demux2/1 -> Demux1/1
  Demux2/2 -> Mux1/8
  Demux/4 -> Mux1/7  "clq"

== system carnot/Storage/Thermal/Ice_Storage ==
  THBsource : Inport
  THBload : Inport  Port=2
  1/h_ice1 : Gain  Gain=1/335e3  SaturateOnIntegerOverflow=on  OutDataTypeStr=Inherit: Same as input  ParamDataTypeStr=Inherit: Same as input
  1/m/cp : Gain  Gain=1/(V_earth*rho_ground*cp_ground)  SaturateOnIntegerOverflow=on  OutDataTypeStr=Inherit: Same as input  ParamDataTypeStr=Inherit: Same as input
  1/vol : Gain  Gain=1/(vol*1e3)  SaturateOnIntegerOverflow=on  OutDataTypeStr=Inherit: Same as input  ParamDataTypeStr=Inherit: Same as input
  Bus Assignment1 : BusAssignment  AssignedSignals=Temperature
  Bus Assignment2 : BusAssignment  AssignedSignals=Temperature
  Bus Creator : BusCreator  Inputs=3
  Bus Creator1 : BusCreator  Inputs=3
  Bus Creator2 : BusCreator  Inputs=3
  Bus Selector1 : BusSelector  OutputSignals=Temperature,MassFlow,Pressure,FluidType,FluidMix
  Bus Selector2 : BusSelector  OutputSignals=Temperature,MassFlow,Pressure,FluidType,FluidMix
  Heat_Exchanger_HP : Subsystem  mask{Lhx=Lhx_hp, Ulen=Ulen_hp, mpc_hp=mpc_hp}
      mask prompts: Lhx "Length of heat exchanger pipe in m"; Ulen "Heat transfer of pipe per length in W/K/m"; mpc_hp "Thermal capacity of pipe per length in J/K/m"
      mask TypeOptions Lhx: Constant/Value
      mask TypeOptions Ulen: U_length/Gain
      mask TypeOptions mpc_hp: Constant1/Value
  Heat_Exchanger_Solar : Subsystem  mask{Lhx=Lhx_sol, Ulen=Ulen_sol, mpc_hp=mpc_sol}
      mask prompts: Lhx "Length of heat exchanger pipe in m"; Ulen "Heat transfer of pipe per length in W/K/m"; mpc_hp "Thermal capacity of pipe per length in J/K/m"
      mask TypeOptions Lhx: Constant/Value
      mask TypeOptions Ulen: U_length/Gain
      mask TypeOptions mpc_hp: Constant1/Value
  Integrator : Integrator  InitialCondition=h_ini
  Integrator1 : Integrator  InitialCondition=4
  Sum1 : Sum  Inputs=+++  SaturateOnIntegerOverflow=on  InputSameDT=on  OutDataTypeStr=Inherit: Same as first input
  Sum2 : Sum  Inputs=-+  SaturateOnIntegerOverflow=on  InputSameDT=on  OutDataTypeStr=Inherit: Same as first input
  Sum3 : Sum  Inputs=-+  SaturateOnIntegerOverflow=on  InputSameDT=on  OutDataTypeStr=Inherit: Same as first input
  Sum4 : Sum  Inputs=-+  SaturateOnIntegerOverflow=on  InputSameDT=on  OutDataTypeStr=Inherit: Same as first input
  T_ground_undisturbed : Subsystem
  TiceCalc2Tice : Lookup  InputValues=[-10 -3 0 10]  Table=[-10 0 0 10]
  UAearth : Gain  Gain=U_earth * A_earth  SaturateOnIntegerOverflow=on  OutDataTypeStr=Inherit: Same as input  ParamDataTypeStr=Inherit: Same as input
  UAtank : Gain  Gain=UA_tank  SaturateOnIntegerOverflow=on  OutDataTypeStr=Inherit: Same as input  ParamDataTypeStr=Inherit: Same as input
  h 2 T : Lookup  InputValues=[-2060*10 -2060*3 335e3 335e3+4182*10]  Table=[-10 -3 0 10]
  THB_source : Outport
  THB_load : Outport  Port=2
  data_IceST : Outport  Port=3
  wires:
  TiceCalc2Tice/1 -> Bus Creator2/1  "Tice"
  Heat_Exchanger_HP/2(Thx) -> Bus Assignment2/2
  Bus Assignment2/1 -> THB_load/1
  Bus Selector2/1 -> Heat_Exchanger_HP/2(Tin)  "<Temperature>"
  Bus Selector2/3 -> Heat_Exchanger_HP/4(p)  "<Pressure>"
  Bus Selector2/5 -> Heat_Exchanger_HP/6(mix)  "<FluidMix>"
  Bus Selector2/2 -> Heat_Exchanger_HP/3(mdot)  "<MassFlow>"
  Bus Selector2/4 -> Heat_Exchanger_HP/5(fluid)  "<FluidType>"
  Bus Selector1/2 -> Heat_Exchanger_Solar/3(mdot)  "<MassFlow>"
  Bus Selector1/4 -> Heat_Exchanger_Solar/5(fluid)  "<FluidType>"
  Bus Selector1/5 -> Heat_Exchanger_Solar/6(mix)  "<FluidMix>"
  Bus Selector1/3 -> Heat_Exchanger_Solar/4(p)  "<Pressure>"
  Bus Selector1/1 -> Heat_Exchanger_Solar/2(Tin)  "<Temperature>"
  Bus Assignment1/1 -> THB_source/1
  Bus Creator2/1 -> Bus Creator1/3  "T"
  T_ground_undisturbed/1(Tearth) -> Bus Creator2/3, Sum3/2  "Tground_far"
  1/h_ice1/1 -> Bus Creator1/2  "SOC"
  Bus Creator1/1 -> data_IceST/1
  THBsource/1 -> Bus Selector1/1, Bus Assignment1/1
  Heat_Exchanger_Solar/2(Thx) -> Bus Assignment1/2
  1/vol/1 -> Integrator/1
  Sum1/1 -> 1/vol/1
  Sum2/1 -> UAtank/1
  UAtank/1 -> Sum1/2, Sum4/1, Bus Creator/2  "Qdot_earth2ice"
  Integrator/1 -> 1/h_ice1/1, h 2 T/1  "h"
  Sum3/1 -> UAearth/1
  UAearth/1 -> Sum4/2
  Sum4/1 -> 1/m/cp/1
  1/m/cp/1 -> Integrator1/1
  Integrator1/1 -> Sum3/1, Sum2/2, Bus Creator2/2  "Tground_close"
  h 2 T/1 -> TiceCalc2Tice/1, Heat_Exchanger_HP/1(Tice), Sum2/1, Heat_Exchanger_Solar/1(Tice)  "TiceCalc"
  Heat_Exchanger_Solar/1(Qdot2ice) -> Bus Creator/3, Sum1/3  "Qdot_from_source"
  THBload/1 -> Bus Selector2/1, Bus Assignment2/1
  Heat_Exchanger_HP/1(Qdot2ice) -> Bus Creator/1, Sum1/1  "Qdot_to_load"
  Bus Creator/1 -> Bus Creator1/1  "Qdot"
